simulink model "Ex_1_4_Control_Puma_2019a"  (R2019a)
settings: Solver=FixedStepAuto  StartTime=0.0  StopTime=6  FixedStep=0.01  RelTol=1e-3
libraries: simulink x6
(part 2 of 2)

== matlab function Ex_1_4_Control_Puma_2019a/Inverse ==
  data: dx input; dy input; dz input; dro input; dpitch input; dyaw input; t1o output; t2o output; t3o output; t4o output; t5o output; t6o output; t1 input; t2 input; t3 input; t4 input; t5 input; t6 input
function [t1o, t2o, t3o, t4o, t5o, t6o]   = Inverse(dx,dy,dz, dro, dpitch, dyaw, t1, t2, t3, t4, t5, t6)

% % dx = dx*0.1;
% % dy = dy*0.1;
% % dz = dz*0.1;
% dro = dro*0.005;
% dpitch = dpitch*1;
% dyaw = dyaw*0.1;

J = [
(cos(t5)*(cos(t2)*sin(t1)*sin(t3) + cos(t3)*sin(t1)*sin(t2)))/10 - (2159*cos(t2)*sin(t1))/5000 - (sin(t5)*(cos(t1)*sin(t4) + cos(t4)*(sin(t1)*sin(t2)*sin(t3) - cos(t2)*cos(t3)*sin(t1))))/10 - (3*cos(t1))/20 + (2159*cos(t2)*sin(t1)*sin(t3))/5000 + (2159*cos(t3)*sin(t1)*sin(t2))/5000 + (203*sin(t1)*sin(t2)*sin(t3))/10000 - (203*cos(t2)*cos(t3)*sin(t1))/10000, (cos(t5)*(cos(t1)*sin(t2)*sin(t3) - cos(t1)*cos(t2)*cos(t3)))/10 - (2159*cos(t1)*sin(t2))/5000 + (2159*cos(t1)*sin(t2)*sin(t3))/5000 + (cos(t4)*sin(t5)*(cos(t1)*cos(t2)*sin(t3) + cos(t1)*cos(t3)*sin(t2)))/10 - (2159*cos(t1)*cos(t2)*cos(t3))/5000 - (203*cos(t1)*cos(t2)*sin(t3))/10000 - (203*cos(t1)*cos(t3)*sin(t2))/10000, (cos(t5)*(cos(t1)*sin(t2)*sin(t3) - cos(t1)*cos(t2)*cos(t3)))/10 + (2159*cos(t1)*sin(t2)*sin(t3))/5000 + (cos(t4)*sin(t5)*(cos(t1)*cos(t2)*sin(t3) + cos(t1)*cos(t3)*sin(t2)))/10 - (2159*cos(t1)*cos(t2)*cos(t3))/5000 - (203*cos(t1)*cos(t2)*sin(t3))/10000 - (203*cos(t1)*cos(t3)*sin(t2))/10000, -(sin(t5)*(cos(t4)*sin(t1) + sin(t4)*(cos(t1)*sin(t2)*sin(t3) - cos(t1)*cos(t2)*cos(t3))))/10, (sin(t5)*(cos(t1)*cos(t2)*sin(t3) + cos(t1)*cos(t3)*sin(t2)))/10 - (cos(t5)*(sin(t1)*sin(t4) - cos(t4)*(cos(t1)*sin(t2)*sin(t3) - cos(t1)*cos(t2)*cos(t3))))/10,                                                                                                                                                       0;
(2159*cos(t1)*cos(t2))/5000 - (3*sin(t1))/20 - (sin(t5)*(sin(t1)*sin(t4) - cos(t4)*(cos(t1)*sin(t2)*sin(t3) - cos(t1)*cos(t2)*cos(t3))))/10 - (cos(t5)*(cos(t1)*cos(t2)*sin(t3) + cos(t1)*cos(t3)*sin(t2)))/10 - (203*cos(t1)*sin(t2)*sin(t3))/10000 + (203*cos(t1)*cos(t2)*cos(t3))/10000 - (2159*cos(t1)*cos(t2)*sin(t3))/5000 - (2159*cos(t1)*cos(t3)*sin(t2))/5000, (cos(t5)*(sin(t1)*sin(t2)*sin(t3) - cos(t2)*cos(t3)*sin(t1)))/10 - (2159*sin(t1)*sin(t2))/5000 - (203*cos(t2)*sin(t1)*sin(t3))/10000 - (203*cos(t3)*sin(t1)*sin(t2))/10000 + (2159*sin(t1)*sin(t2)*sin(t3))/5000 + (cos(t4)*sin(t5)*(cos(t2)*sin(t1)*sin(t3) + cos(t3)*sin(t1)*sin(t2)))/10 - (2159*cos(t2)*cos(t3)*sin(t1))/5000, (cos(t5)*(sin(t1)*sin(t2)*sin(t3) - cos(t2)*cos(t3)*sin(t1)))/10 - (203*cos(t2)*sin(t1)*sin(t3))/10000 - (203*cos(t3)*sin(t1)*sin(t2))/10000 + (2159*sin(t1)*sin(t2)*sin(t3))/5000 + (cos(t4)*sin(t5)*(cos(t2)*sin(t1)*sin(t3) + cos(t3)*sin(t1)*sin(t2)))/10 - (2159*cos(t2)*cos(t3)*sin(t1))/5000,  (sin(t5)*(cos(t1)*cos(t4) - sin(t4)*(sin(t1)*sin(t2)*sin(t3) - cos(t2)*cos(t3)*sin(t1))))/10, (cos(t5)*(cos(t1)*sin(t4) + cos(t4)*(sin(t1)*sin(t2)*sin(t3) - cos(t2)*cos(t3)*sin(t1))))/10 + (sin(t5)*(cos(t2)*sin(t1)*sin(t3) + cos(t3)*sin(t1)*sin(t2)))/10,                                                                                                                                                       0;
                                                                                                                                                                                                                                                                                                                                                                     0,                                                                         (2159*cos(t2)*sin(t3))/5000 - (203*cos(t2)*cos(t3))/10000 - (2159*cos(t2))/5000 + (2159*cos(t3)*sin(t2))/5000 + (203*sin(t2)*sin(t3))/10000 + (cos(t5)*(cos(t2)*sin(t3) + cos(t3)*sin(t2)))/10 + (cos(t4)*sin(t5)*(cos(t2)*cos(t3) - sin(t2)*sin(t3)))/10,                                                                 (2159*cos(t2)*sin(t3))/5000 - (203*cos(t2)*cos(t3))/10000 + (2159*cos(t3)*sin(t2))/5000 + (203*sin(t2)*sin(t3))/10000 + (cos(t5)*(cos(t2)*sin(t3) + cos(t3)*sin(t2)))/10 + (cos(t4)*sin(t5)*(cos(t2)*cos(t3) - sin(t2)*sin(t3)))/10,                                     -(sin(t4)*sin(t5)*(cos(t2)*sin(t3) + cos(t3)*sin(t2)))/10,                                                     (sin(t5)*(cos(t2)*cos(t3) - sin(t2)*sin(t3)))/10 + (cos(t4)*cos(t5)*(cos(t2)*sin(t3) + cos(t3)*sin(t2)))/10,                                                                                                                                                       0;
                                                                                                                                                                                                                                                                                                                                                                     0,                                                                                                                                                                                                                                                                                                                          -sin(t1),                                                                                                                                                                                                                                                                                            -sin(t1),                                           - cos(t1)*cos(t2)*sin(t3) - cos(t1)*cos(t3)*sin(t2),                                                                                 - cos(t4)*sin(t1) - sin(t4)*(cos(t1)*sin(t2)*sin(t3) - cos(t1)*cos(t2)*cos(t3)), - sin(t5)*(sin(t1)*sin(t4) - cos(t4)*(cos(t1)*sin(t2)*sin(t3) - cos(t1)*cos(t2)*cos(t3))) - cos(t5)*(cos(t1)*cos(t2)*sin(t3) + cos(t1)*cos(t3)*sin(t2));
                                                                                                                                                                                                                                                                                                                                                                     0,                                                                                                                                                                                                                                                                                                                           cos(t1),                                                                                                                                                                                                                                                                                             cos(t1),                                           - cos(t2)*sin(t1)*sin(t3) - cos(t3)*sin(t1)*sin(t2),                                                                                   cos(t1)*cos(t4) - sin(t4)*(sin(t1)*sin(t2)*sin(t3) - cos(t2)*cos(t3)*sin(t1)),   sin(t5)*(cos(t1)*sin(t4) + cos(t4)*(sin(t1)*sin(t2)*sin(t3) - cos(t2)*cos(t3)*sin(t1))) - cos(t5)*(cos(t2)*sin(t1)*sin(t3) + cos(t3)*sin(t1)*sin(t2));
                                                                                                                                                                                                                                                                                                                                                                     1,                                                                                                                                                                                                                                                                                                                                 0,                                                                                                                                                                                                                                                                                                   0,                                                             sin(t2)*sin(t3) - cos(t2)*cos(t3),                                                                                                                    -sin(t4)*(cos(t2)*sin(t3) + cos(t3)*sin(t2)),                                                       cos(t4)*sin(t5)*(cos(t2)*sin(t3) + cos(t3)*sin(t2)) - cos(t5)*(cos(t2)*cos(t3) - sin(t2)*sin(t3));];

small_const = 0.1;
if det(J) == 0
    J = J + diag(small_const);
end

res = J\[dx; dy; dz; dro; dpitch; dyaw];
dt1_ = res(1,1);
dt2_ = res(2,1);
dt3_ = res(3,1);
dt4_ = res(4,1);
dt5_ = res(5,1);
dt6_ = res(6,1);

damp = 0.1;
t1 = t1 + damp*dt1_;
t2 = t2 + damp*dt2_;
t3 = t3 + damp*dt3_;
t4 = t4 + damp*dt4_; 
t5 = t5 + damp*dt5_;
t6 = t6 + damp*dt6_;

t1o = t1; 
t2o = t2; 
t3o = t3; 
t4o = t4; 
t5o = t5; 
t6o = t6; 

end
